simulink model "poleplacemente_cicloaperto_WP2"  (R2023a)
settings: Solver=VariableStepAuto  StartTime=0.0  StopTime=10.0  RelTol=1e-3
values from neighbouring files (symbols this model uses):
  A = [0 1; 9.81 -0.1]    [WP2.m]    (also in poleplacement_WP2.m; poleplacement_test1_WP2.m; poleplacement_test2_WP2.m; poleplacement_test3_WP2.m)
  B = [0; 1]    [WP2.m]    (also in poleplacement_WP2.m; poleplacement_test1_WP2.m; poleplacement_test2_WP2.m; poleplacement_test3_WP2.m)
  K = [k1 k2]    [WP2.m]    (also in parameters_for_equipollenza_WP2.m = [8109.81 179.9]; poleplacement_WP2.m = [1609.81 39.90]; poleplacement_test1_WP2.m = [739.81 53.9]; poleplacement_test2_WP2.m = [17.1 5.3])
  k_r = -1/(C*inv(A-B*K)*B)    [poleplacement_WP2.m]    (also in poleplacement_test1_WP2.m; poleplacement_test2_WP2.m; poleplacement_test3_WP2.m; poleplacement_test4_WP2.m)
settings Model: Creator=miche  LastModifiedBy=miche

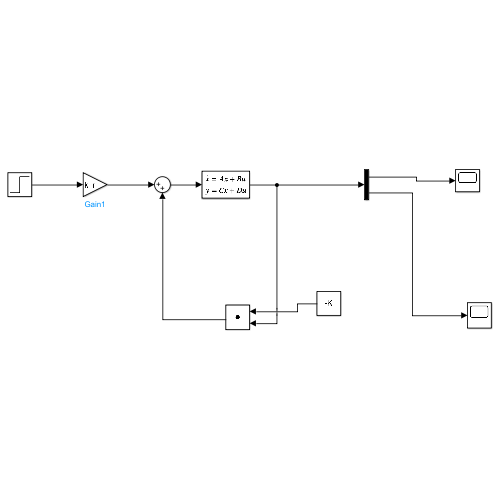
[thumbnail: Simulink's stored preview of the top-level diagram]
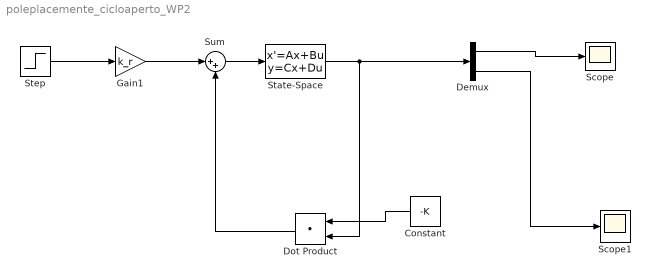
== system poleplacemente_cicloaperto_WP2 ==
  Constant : Constant  Value=-K
  Demux : Demux  Outputs=2
  Dot Product : DotProduct  OutDataTypeStr=Inherit: Inherit via internal rule
  Gain1 : Gain  Gain=k_r
  Scope : Scope
  Scope1 : Scope
  State-Space : StateSpace  A=A  B=B  C=eye(2)  D=[0;0]  InitialCondition=[0,0]
  Step : Step  After=pi  SampleTime=0
  Sum : Sum  Inputs=|++
  wires:
  Dot Product/1 -> Sum/2
  Demux/1 -> Scope/1
  Demux/2 -> Scope1/1
  Constant/1 -> Dot Product/1
  State-Space/1 -> Dot Product/2, Demux/1
  Step/1 -> Gain1/1
  Gain1/1 -> Sum/1
  Sum/1 -> State-Space/1
